simulink model "TEST_AccHitGround"  (R2020b)
settings: Solver=ode1  StartTime=0.0  StopTime=tspan(2)  FixedStep=SimParam.Navi.Ts_Base  RelTol=1e-3
undefined symbols (not defined in the file or in its folder): IN_SENSOR_SIM
settings Model: PauseTimes=880  Creator=sl  LastModifiedBy=sl
settings DataIOCC: SaveOutput=off  SaveTime=off
settings OptimizationCC: DefaultParameterBehavior=Inlined  EnhancedBackFolding=on  PassReuseOutputArgsAs=Individual arguments  ZeroExternalMemoryAtStartup=off  ZeroInternalMemoryAtStartup=off  OptimizeBlockOrder=speed  DifferentSizesBufferReuse=on  OptimizationCustomize=off  EfficientTunableParamExpr=on
settings DebuggingCC: InheritedTsInSrcMsg=none  ParameterPrecisionLossMsg=none  ParameterTunabilityLossMsg=error  UnconnectedInputMsg=none  UnconnectedOutputMsg=none  UnconnectedLineMsg=none
settings HardwareCC: ProdBitPerPointer=32  ProdBitPerSizeT=32  ProdBitPerPtrDiffT=32  ProdLargestAtomicInteger=Long  ProdLargestAtomicFloat=Double  ProdWordSize=32  ProdHWDeviceType=ARM Compatible->ARM Cortex
settings ModelReferenceCC: ModelReferenceNumInstancesAllowed=Single
settings SFSimCC: MATLABDynamicMemAlloc=off
settings RTWCC: Description=Embedded Coder  SystemTargetFile=ert.tlc  TemplateMakefile=ert_default_tmf  GenerateReport=on  IncludeHyperlinkInReport=on  LaunchReport=on  GenerateTraceInfo=on  GenerateTraceReport=on  GenerateTraceReportSl=on  GenerateTraceReportSf=on  GenerateTraceReportEml=on
settings CodeAppCC: ForceParamTrailComments=on  IgnoreCustomStorageClasses=off  MaxIdLength=48  OperatorAnnotations=on  SimulinkDataObjDesc=on  SFDataObjDesc=on  InsertBlockDesc=on
settings ERTTargetCC: TargetLangStandard=C99 (ISO)  GenerateSampleERTMain=on  LogVarNameModifier=none  SupportVariableSizeSignals=on  InlinedParameterPlacement=NonHierarchical  ERTCustomFileTemplate=example_file_process.tlc

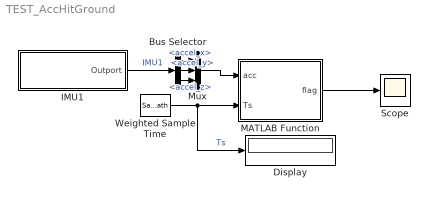
== system TEST_AccHitGround ==
  Bus Selector : BusSelector  OutputSignals=accel_x,accel_y,accel_z
  Display : Display
  IMU1 : Subsystem  mask{data=IN_SENSOR_SIM.IMU1}
      mask prompts: data "IMU数据结构体"
  MATLAB Function : MATLAB Function  TreatAsAtomicUnit=on
  Mux : Mux  Inputs=3
  Scope : Scope
  Weighted Sample Time : SampleTimeMath  TsampMathOp=Ts Only
  wires:
  IMU1/1(Outport) -> Bus Selector/1  "IMU1"
  Weighted Sample Time/1 -> Display/1, MATLAB Function/2(Ts)  "Ts"
  MATLAB Function/1(flag) -> Scope/1
  Bus Selector/1 -> Mux/1  "<accel_x>"
  Bus Selector/2 -> Mux/2  "<accel_y>"
  Bus Selector/3 -> Mux/3  "<accel_z>"
  Mux/1 -> MATLAB Function/1(acc)

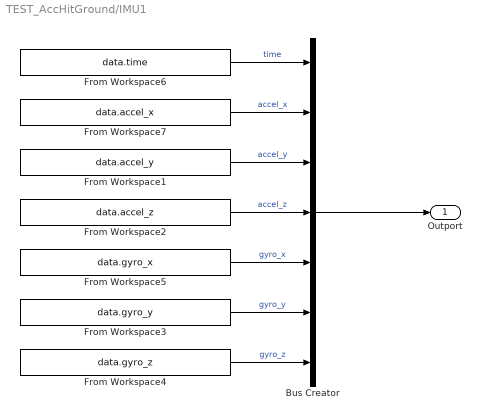
== system TEST_AccHitGround/IMU1 ==
  Bus Creator : BusCreator  Inputs=7
  From Workspace1 : FromWorkspace  VariableName=data.accel_y  OutputAfterFinalValue=Holding final value
  From Workspace2 : FromWorkspace  VariableName=data.accel_z  OutputAfterFinalValue=Holding final value
  From Workspace3 : FromWorkspace  VariableName=data.gyro_y  OutputAfterFinalValue=Holding final value
  From Workspace4 : FromWorkspace  VariableName=data.gyro_z  OutputAfterFinalValue=Holding final value
  From Workspace5 : FromWorkspace  VariableName=data.gyro_x  OutputAfterFinalValue=Holding final value
  From Workspace6 : FromWorkspace  VariableName=data.time  OutputAfterFinalValue=Holding final value
  From Workspace7 : FromWorkspace  VariableName=data.accel_x  OutputAfterFinalValue=Holding final value
  Outport : Outport
  wires:
  From Workspace1/1 -> Bus Creator/3  "accel_y"
  From Workspace4/1 -> Bus Creator/7  "gyro_z"
  Bus Creator/1 -> Outport/1
  From Workspace2/1 -> Bus Creator/4  "accel_z"
  From Workspace5/1 -> Bus Creator/5  "gyro_x"
  From Workspace7/1 -> Bus Creator/2  "accel_x"
  From Workspace6/1 -> Bus Creator/1  "time"
  From Workspace3/1 -> Bus Creator/6  "gyro_y"

== matlab function TEST_AccHitGround/MATLAB Function ==
  data: acc input; flag output; Ts input
function flag = fcn(acc, Ts)
persistent duration
if isempty(duration)
    duration = 0;
end
hitSuccess = acc(3)>15;
flag = true;
if not( hitSuccess ) 
    duration = duration + Ts;
    if duration > 0.5 % 没有出现大az一段时间后,false
        flag = false;
    end 
else % 出现大az，true
    flag = true;
    duration = 0;
end
